simulink model "robot1"  (R2016b)
settings: Solver=FixedStepAuto  StartTime=0.0  StopTime=30  FixedStep=0.005  RelTol=1e-3
settings Model: Creator=赵安  LastModifiedBy=赵安

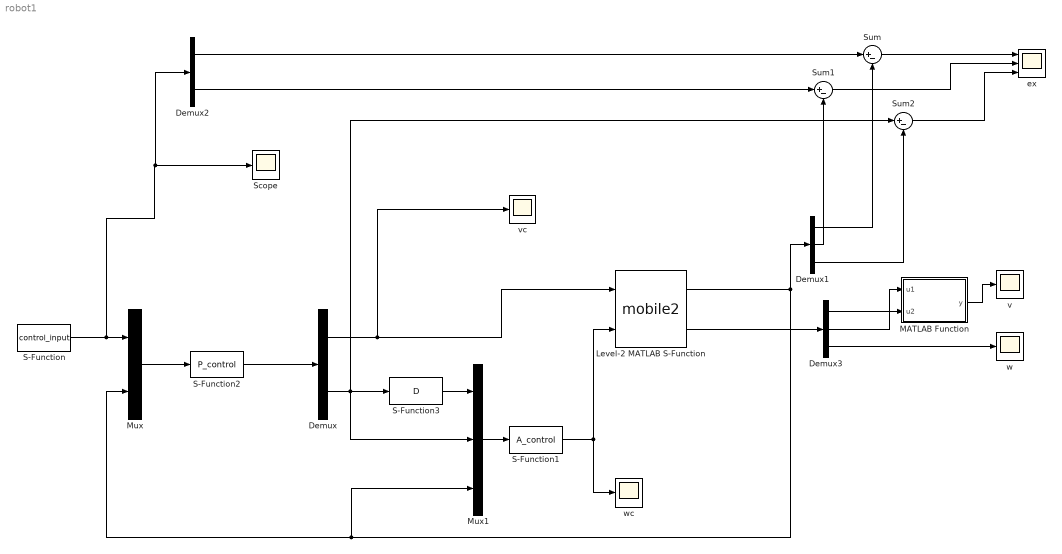
== system robot1 ==
  Demux : Demux  Outputs=2
  Demux1 : Demux  Outputs=3
  Demux2 : Demux  Outputs=2
  Demux3 : Demux  Outputs=3
  Level-2 MATLAB S-Function : M-S-Function  FunctionName=mobile2
  MATLAB Function : MATLAB Function  TreatAsAtomicUnit=on
  Mux : Mux  Inputs=2
  Mux1 : Mux  Inputs=3
  S-Function : S-Function  FunctionName=control_input  SFunctionDeploymentMode=off  EnableBusSupport=off
  S-Function1 : S-Function  FunctionName=A_control  SFunctionDeploymentMode=off  EnableBusSupport=off
  S-Function2 : S-Function  FunctionName=P_control  SFunctionDeploymentMode=off  EnableBusSupport=off
  S-Function3 : S-Function  FunctionName=D  SFunctionDeploymentMode=off  EnableBusSupport=off
  Scope : Scope
  Sum : Sum  Inputs=|+-
  Sum1 : Sum  Inputs=|+-
  Sum2 : Sum  Inputs=|+-
  ex : Scope  NumInputPorts=3
  "v " : Scope
  "vc " : Scope
  w : Scope
  "wc " : Scope
  wires:
  S-Function/1 -> Demux2/1, Scope/1, Mux/1
  Mux/1 -> S-Function2/1
  S-Function2/1 -> Demux/1
  Demux/2 -> Mux1/2, S-Function3/1, Sum2/1
  S-Function3/1 -> Mux1/1
  Mux1/1 -> S-Function1/1
  Level-2 MATLAB S-Function/1 -> Mux/2, Mux1/3, Demux1/1
  Demux1/1 -> Sum/2
  Demux1/2 -> Sum1/2
  Demux2/1 -> Sum/1
  Demux2/2 -> Sum1/1
  Sum/1 -> ex/1
  Demux1/3 -> Sum2/2
  Level-2 MATLAB S-Function/2 -> Demux3/1
  Demux3/3 -> w/1
  Demux3/1 -> MATLAB Function/1(u1)
  Demux3/2 -> MATLAB Function/2(u2)
  MATLAB Function/1(y) -> "v "/1
  Demux/1 -> Level-2 MATLAB S-Function/1, "vc "/1
  S-Function1/1 -> Level-2 MATLAB S-Function/2, "wc "/1
  Sum1/1 -> ex/2
  Sum2/1 -> ex/3

== matlab function robot1/MATLAB Function ==
  data: u1 input; y output; u2 input
function y = fcn(u1,u2)

y = sqrt(u1^2+u2^2);
